simulink model "SET2"  (Simulink 5.0)
settings: Solver=ode45  StartTime=0.0  StopTime=10.0  RelTol=1e-3
settings Model: LastModifiedBy=Administrator

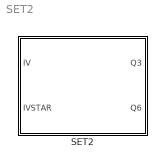
== system SET2 ==
  SET2 : Stateflow chart

== stateflow chart SET2 ==
  settings: updateMethod=CONTINUOUS  executeAtInitialization=1
  state B/
    state B1/
      during:Q3=1;Q6=0;
    state B2/
      during:Q6=1;Q3=0;
    B1 -> B2 : [IV>IVSTAR]
    B2 -> B1 : [IV<IVSTAR]
    (default) -> B1 : [1]
  (default) -> B : [1]
  data: IV input double; IVSTAR input double; Q3 output double; Q6 output double
